simulink model "Ejercicio1"  (R2024a)
settings: Solver=ode1  StartTime=0.0  StopTime=10.0  FixedStep=0.001  RelTol=1e-3
undefined symbols (not defined in the file): d, ki, kp
settings Model: Creator=richie  LastModifiedBy=richie

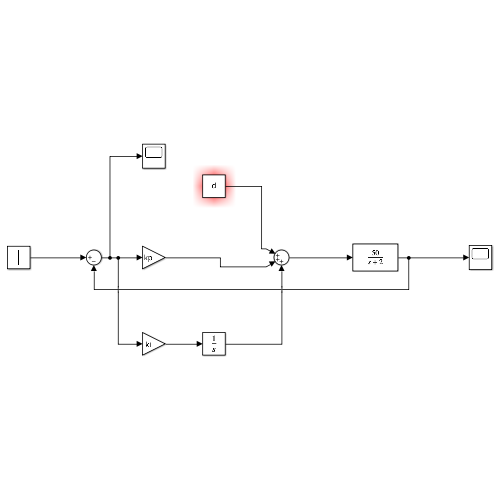
[thumbnail: Simulink's stored preview of the top-level diagram]
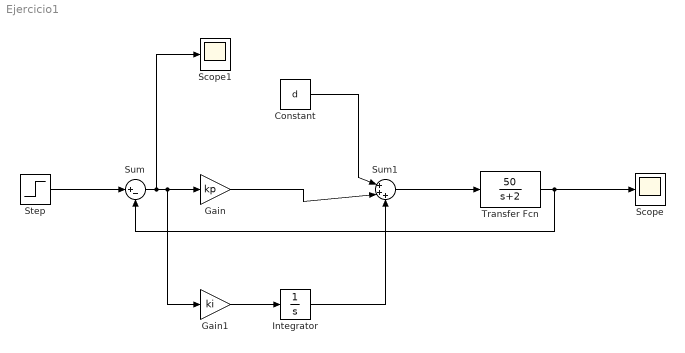
== system Ejercicio1 ==
  Constant : Constant  Value=d
  Gain : Gain  Gain=kp
  Gain1 : Gain  Gain=ki
  Integrator : Integrator
  Scope : Scope
  Scope1 : Scope
  Step : Step  SampleTime=0
  Sum : Sum  Inputs=|+-
  Sum1 : Sum  Inputs=|+++
  Transfer Fcn : TransferFcn  Numerator=[50]  Denominator=[1 2]
  wires:
  Sum1/1 -> Transfer Fcn/1
  Gain1/1 -> Integrator/1
  Sum/1 -> Scope1/1, Gain1/1, Gain/1
  Step/1 -> Sum/1
  Transfer Fcn/1 -> Scope/1, Sum/2
  Integrator/1 -> Sum1/3
  Gain/1 -> Sum1/2
  Constant/1 -> Sum1/1
